simulink model "Dynamic_Phasor_Extraction_Moving_Average"  (R2021b)
settings: Solver=VariableStepAuto  StartTime=0.0  StopTime=10.0  RelTol=1e-3
undefined symbols (not defined in the file): Ts
libraries: eeGeneralControl x3, spsFourierLib x3
settings Model: Creator=Antero  LastModifiedBy=Antero

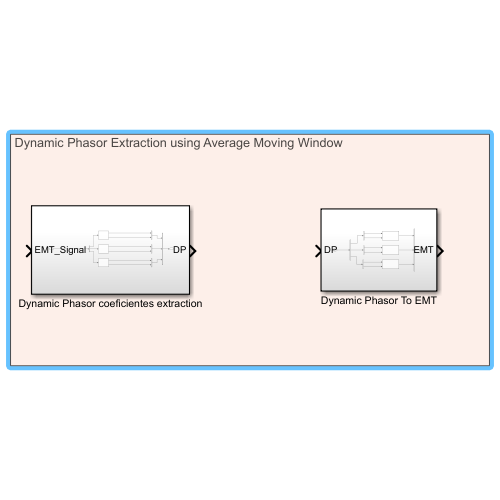
[thumbnail: Simulink's stored preview of the top-level diagram]
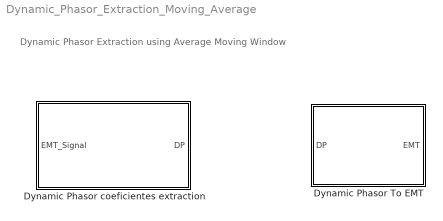
== system Dynamic_Phasor_Extraction_Moving_Average ==
  note: Dynamic Phasor Extraction using Average Moving Window
  Dynamic Phasor To EMT : Subsystem
  Dynamic Phasor coeficientes extraction : Subsystem

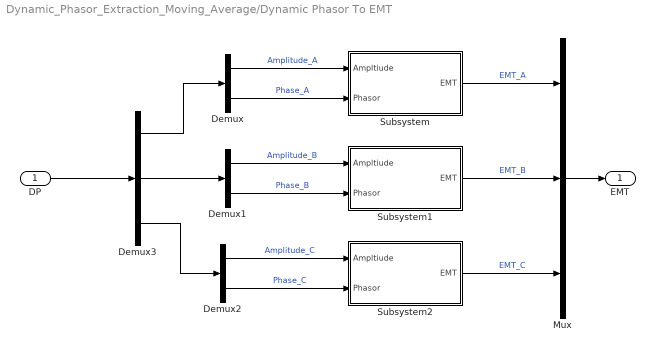
== system Dynamic_Phasor_Extraction_Moving_Average/Dynamic Phasor To EMT ==
  DP : Inport
  Demux : Demux  Outputs=2
  Demux1 : Demux  Outputs=2
  Demux2 : Demux  Outputs=2
  Demux3 : Demux  Outputs=3
  Mux : Mux  Inputs=3
  Subsystem : Subsystem
  Subsystem1 : Subsystem
  Subsystem2 : Subsystem
  EMT : Outport
  wires:
  Subsystem2/1(EMT) -> Mux/3  "EMT_C"
  Subsystem1/1(EMT) -> Mux/2  "EMT_B"
  Demux/1 -> Subsystem/1(Ampltiude)  "Amplitude_A"
  Demux/2 -> Subsystem/2(Phasor)  "Phase_A"
  Demux1/1 -> Subsystem1/1(Ampltiude)  "Amplitude_B"
  Demux1/2 -> Subsystem1/2(Phasor)  "Phase_B"
  Demux2/1 -> Subsystem2/1(Ampltiude)  "Amplitude_C"
  Demux2/2 -> Subsystem2/2(Phasor)  "Phase_C"
  Subsystem/1(EMT) -> Mux/1  "EMT_A"
  Mux/1 -> EMT/1
  DP/1 -> Demux3/1
  Demux3/1 -> Demux/1
  Demux3/2 -> Demux1/1
  Demux3/3 -> Demux2/1

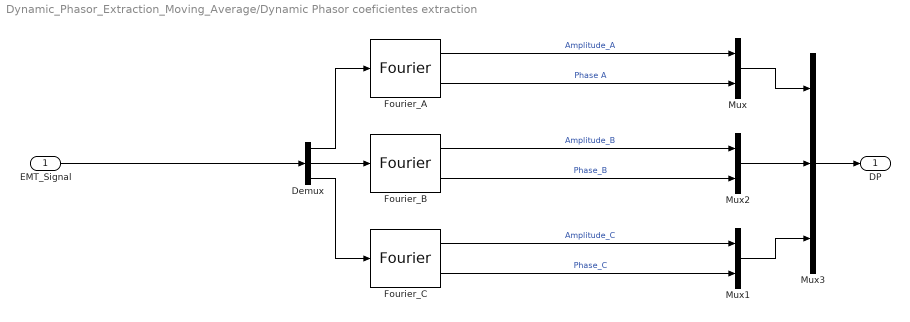
== system Dynamic_Phasor_Extraction_Moving_Average/Dynamic Phasor coeficientes extraction ==
  EMT_Signal : Inport
  Demux : Demux  Outputs=3
  Fourier_A : spsFourierLib/Fourier  Freq=60  n=1  InInit=[1,0]  Ts=Ts
      settings: SourceProductBaseCode=PS
  Fourier_B : spsFourierLib/Fourier  Freq=60  n=1  InInit=[1,-120 ]  Ts=Ts
      settings: SourceProductBaseCode=PS
  Fourier_C : spsFourierLib/Fourier  Freq=60  n=1  InInit=[1,+120 ]  Ts=Ts
      settings: SourceProductBaseCode=PS
  Mux : Mux  Inputs=2
  Mux1 : Mux  Inputs=2
  Mux2 : Mux  Inputs=2
  Mux3 : Mux  Inputs=3
  DP : Outport
  wires:
  Demux/2 -> Fourier_B/1
  Fourier_B/2 -> Mux2/2  "Phase_B"
  Demux/3 -> Fourier_C/1
  Demux/1 -> Fourier_A/1
  Fourier_C/1 -> Mux1/1  "Amplitude_C"
  EMT_Signal/1 -> Demux/1
  Fourier_C/2 -> Mux1/2  "Phase_C"
  Fourier_A/1 -> Mux/1  "Amplitude_A"
  Fourier_A/2 -> Mux/2  "Phase A"
  Fourier_B/1 -> Mux2/1  "Amplitude_B"
  Mux2/1 -> Mux3/2
  Mux1/1 -> Mux3/3
  Mux/1 -> Mux3/1
  Mux3/1 -> DP/1

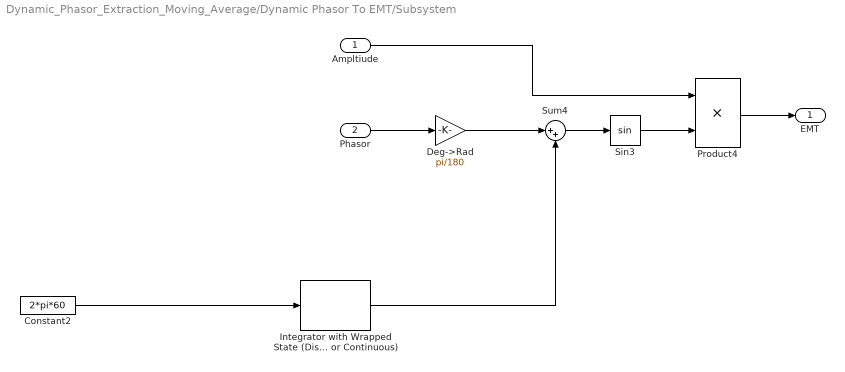
== system Dynamic_Phasor_Extraction_Moving_Average/Dynamic Phasor To EMT/Subsystem ==
  Ampltiude : Inport
  Phasor : Inport  Port=2
  Constant2 : Constant  Value=2*pi*60
  Deg->Rad : Gain  Gain=pi/180
  Integrator with Wrapped State (Discrete or Continuous) : eeGeneralControl/Integrator with Wrapped State (Discrete or Continuous)  LabelModeActiveChoice=Discrete  WrappedStateUpperValue=2*pi  WrappedStateLowerValue=0  x0=0  Ts=-1
      settings: SourceProductBaseCode=PS
  Product4 : Product
  Sin3 : Trigonometry
  Sum4 : Sum  Inputs=|++
  EMT : Outport
  wires:
  Product4/1 -> EMT/1
  Ampltiude/1 -> Product4/1
  Integrator with Wrapped State (Discrete or Continuous)/1 -> Sum4/2
  Phasor/1 -> Deg->Rad/1
  Sum4/1 -> Sin3/1
  Sin3/1 -> Product4/2
  Constant2/1 -> Integrator with Wrapped State (Discrete or Continuous)/1
  Deg->Rad/1 -> Sum4/1

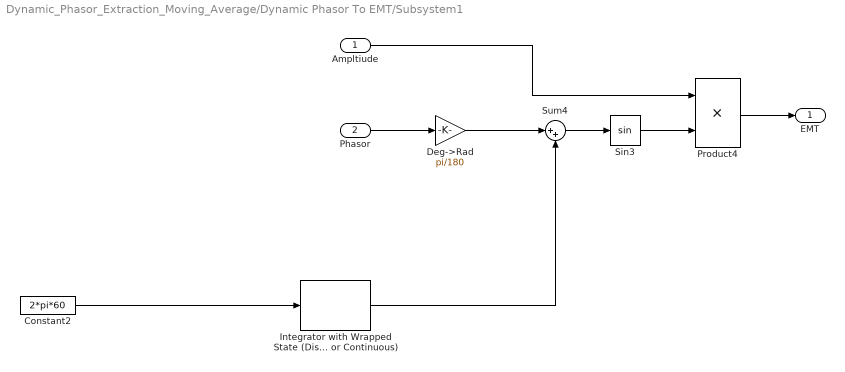
== system Dynamic_Phasor_Extraction_Moving_Average/Dynamic Phasor To EMT/Subsystem1 ==
  Ampltiude : Inport
  Phasor : Inport  Port=2
  Constant2 : Constant  Value=2*pi*60
  Deg->Rad : Gain  Gain=pi/180
  Integrator with Wrapped State (Discrete or Continuous) : eeGeneralControl/Integrator with Wrapped State (Discrete or Continuous)  LabelModeActiveChoice=Discrete  WrappedStateUpperValue=2*pi  WrappedStateLowerValue=0  x0=0  Ts=-1
      settings: SourceProductBaseCode=PS
  Product4 : Product
  Sin3 : Trigonometry
  Sum4 : Sum  Inputs=|++
  EMT : Outport
  wires:
  Deg->Rad/1 -> Sum4/1
  Constant2/1 -> Integrator with Wrapped State (Discrete or Continuous)/1
  Sin3/1 -> Product4/2
  Sum4/1 -> Sin3/1
  Phasor/1 -> Deg->Rad/1
  Integrator with Wrapped State (Discrete or Continuous)/1 -> Sum4/2
  Ampltiude/1 -> Product4/1
  Product4/1 -> EMT/1

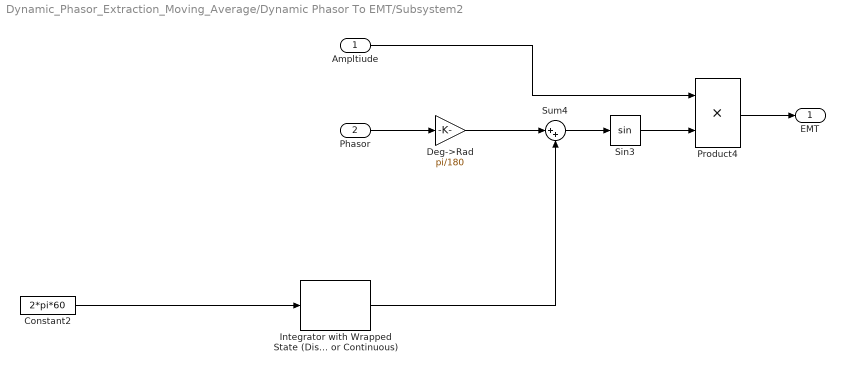
== system Dynamic_Phasor_Extraction_Moving_Average/Dynamic Phasor To EMT/Subsystem2 ==
  Ampltiude : Inport
  Phasor : Inport  Port=2
  Constant2 : Constant  Value=2*pi*60
  Deg->Rad : Gain  Gain=pi/180
  Integrator with Wrapped State (Discrete or Continuous) : eeGeneralControl/Integrator with Wrapped State (Discrete or Continuous)  LabelModeActiveChoice=Discrete  WrappedStateUpperValue=2*pi  WrappedStateLowerValue=0  x0=0  Ts=-1
      settings: SourceProductBaseCode=PS
  Product4 : Product
  Sin3 : Trigonometry
  Sum4 : Sum  Inputs=|++
  EMT : Outport
  wires:
  Product4/1 -> EMT/1
  Ampltiude/1 -> Product4/1
  Integrator with Wrapped State (Discrete or Continuous)/1 -> Sum4/2
  Phasor/1 -> Deg->Rad/1
  Sum4/1 -> Sin3/1
  Sin3/1 -> Product4/2
  Constant2/1 -> Integrator with Wrapped State (Discrete or Continuous)/1
  Deg->Rad/1 -> Sum4/1
